simulink model "Main_System"  (R2024b)
settings: Solver=FixedStepAuto  StartTime=0.0  StopTime=10.0  FixedStep=0.01  RelTol=1e-3
model workspace (MAT data in the model file):
  U2 = Simulink.Parameter
  U2.Value = 1
  U2.Complexity = 'real'
  U2.Dimensions = [1 1]
  U2.DataType = 'auto'
  W = Simulink.Parameter
  W.Value = 10
  W.Complexity = 'real'
  W.Dimensions = [1 1]
  W.DataType = 'auto'
  W1 = Simulink.Parameter
  W1.Value = 8.71893412272
  W1.Complexity = 'real'
  W1.Dimensions = [1 1]
  W1.DataType = 'auto'
  W2 = Simulink.Parameter
  W2.Value = 4.12765808105
  W2.Complexity = 'real'
  W2.Dimensions = [1 1]
  W2.DataType = 'auto'
  mu1 = Simulink.Parameter
  mu1.Value = 0
  mu1.Complexity = 'real'
  mu1.Dimensions = [1 1]
  mu1.DataType = 'auto'
  mu2 = Simulink.Parameter
  mu2.Value = 0
  mu2.Complexity = 'real'
  mu2.Dimensions = [1 1]
  mu2.DataType = 'auto'
  pi = 3.142
  tou = Simulink.Parameter
  tou.Value = 5
  tou.Complexity = 'real'
  tou.Dimensions = [1 1]
  tou.DataType = 'auto'
  tou1 = Simulink.Parameter
  tou1.Value = 4.94300842285
  tou1.Complexity = 'real'
  tou1.Dimensions = [1 1]
  tou1.DataType = 'auto'
  tou2 = Simulink.Parameter
  tou2.Value = 4.95458272298
  tou2.Complexity = 'real'
  tou2.Dimensions = [1 1]
  tou2.DataType = 'auto'
settings Model: Creator=nith  LastModifiedBy=nith

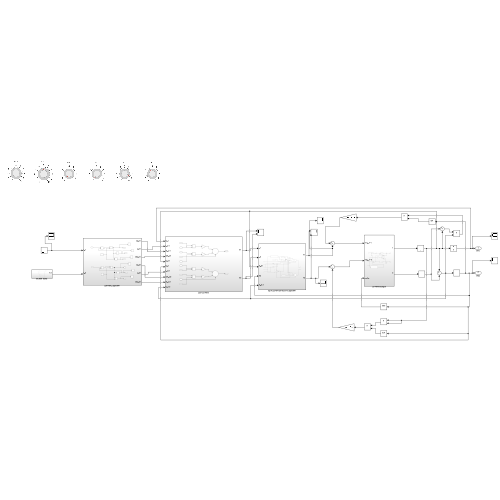
[thumbnail: Simulink's stored preview of the top-level diagram]
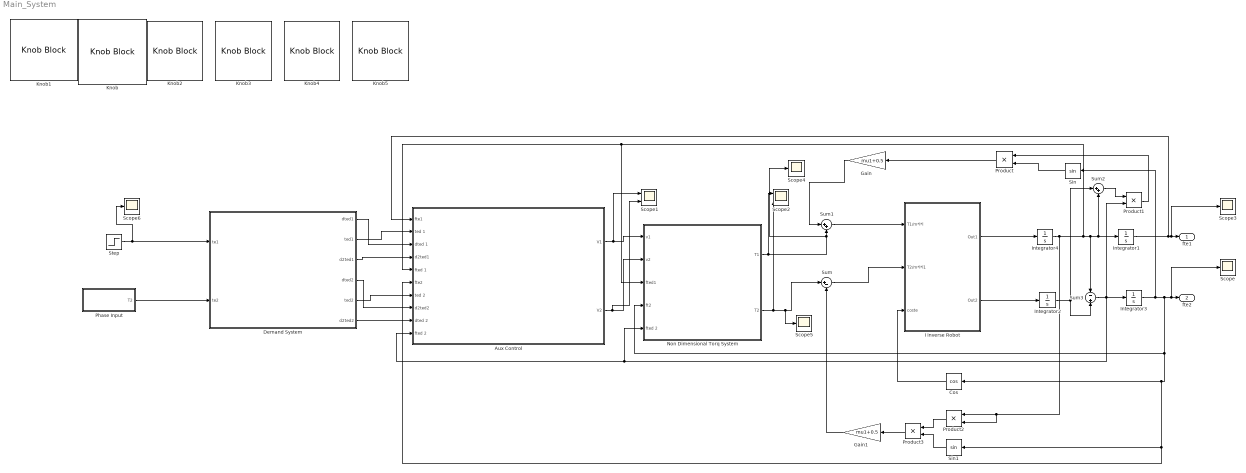
== system Main_System ==
  Aux Control : Subsystem
  Cos : Trigonometry  Operator=cos
  Demand System : Subsystem
  Gain : Gain  Gain=mu1+0.5
  Gain1 : Gain  Gain=mu1+0.5
  I inverse Robot : Subsystem
  Integrator{1..4} (4 alike) : Integrator
  Knob{,1..5} (6 alike) : KnobBlock  ScaleMax=10
  Non Dimensional Torq System : Subsystem
  Phase Input : Subsystem
  Product{,1..3} (4 alike) : Product
  Scope{,3..6} (5 alike) : Scope
  Scope1 : Scope  NumInputPorts=2
  Scope2 : Scope  NumInputPorts=2
  Sin : Trigonometry
  Sin1 : Trigonometry
  Step : Step  Time=0.5  After=6.87*(pi/180)  SampleTime=0
  Sum : Sum  Inputs=|+-
  Sum1 : Sum  Inputs=|++
  Sum2 : Sum  Inputs=|++
  Sum3 : Sum  Inputs=-+
  fte1 : Outport
  fte2 : Outport  Port=2
  wires:
  Demand System/2(ted1) -> Aux Control/2(ted 1)
  Demand System/1(dted1) -> Aux Control/3(dted 1)
  Demand System/3(d2ted1) -> Aux Control/4(d2ted1)
  Demand System/4(dted2) -> Aux Control/8(d2ted2)
  Demand System/5(ted2) -> Aux Control/7(ted 2)
  Demand System/6(d2ted2) -> Aux Control/9(dted 2)
  Integrator4/1 -> Sum3/1, Integrator1/1, Sum2/2, Non Dimensional Torq System/3(fted1), Aux Control/5(fted 1), Product2/2, Product2/1
  Integrator1/1 -> Aux Control/1(fte1), Scope3/1, fte1/1
  Integrator2/1 -> Sum2/1, Sum3/2
  Sum3/1 -> Non Dimensional Torq System/5(fted 2), Aux Control/10(fted 2), Integrator3/1, Product1/2
  Integrator3/1 -> Sin/1, Non Dimensional Torq System/4(ft2), Cos/1, Aux Control/6(fte2), Sin1/1, Scope/1, fte2/1
  Non Dimensional Torq System/1(T1) -> Scope2/1, Scope4/1, Sum1/2
  Non Dimensional Torq System/2(T2) -> Scope5/1, Sum/1, Scope2/2
  Sum1/1 -> I inverse Robot/1(T1/m*l*l)
  Sum/1 -> I inverse Robot/2(T2/m*l*l1)
  Cos/1 -> I inverse Robot/3(coste)
  Product2/1 -> Product3/1
  Sin1/1 -> Product3/2
  Sin/1 -> Product/2
  Product1/1 -> Product/1
  Sum2/1 -> Product1/1
  Aux Control/1(V1) -> Scope1/1, Non Dimensional Torq System/1(v1)
  Aux Control/2(V2) -> Scope1/2, Non Dimensional Torq System/2(v2)
  Product/1 -> Gain/1
  I inverse Robot/1(Out1) -> Integrator4/1
  I inverse Robot/2(Out2) -> Integrator2/1
  Phase Input/1(T2) -> Demand System/2(te2)
  Step/1 -> Scope6/1, Demand System/1(te1)
  Gain/1 -> Sum1/1
  Product3/1 -> Gain1/1
  Gain1/1 -> Sum/2

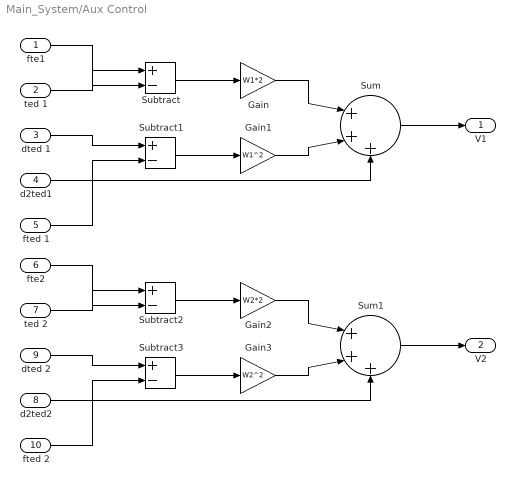
== system Main_System/Aux Control ==
  fte1 : Inport
  ted 1 : Inport  Port=2
  dted 1 : Inport  Port=3
  d2ted1 : Inport  Port=4
  fted 1 : Inport  Port=5
  fte2 : Inport  Port=6
  ted 2 : Inport  Port=7
  d2ted2 : Inport  Port=8
  dted 2 : Inport  Port=9
  fted 2 : Inport  Port=10
  Gain : Gain  Gain=W1*2
  Gain1 : Gain  Gain=W1^2
  Gain2 : Gain  Gain=W2*2
  Gain3 : Gain  Gain=W2^2
  Subtract{,1..3} (4 alike) : Sum  Inputs=+-
  Sum : Sum  Inputs=|+++
  Sum1 : Sum  Inputs=|+++
  V1 : Outport
  V2 : Outport  Port=2
  wires:
  Subtract/1 -> Gain/1
  Gain3/1 -> Sum1/2
  ted 2/1 -> Subtract2/1
  fted 2/1 -> Subtract3/2
  Sum/1 -> V1/1
  Sum1/1 -> V2/1
  dted 2/1 -> Subtract3/1
  fte1/1 -> Subtract/2
  Subtract3/1 -> Gain3/1
  d2ted1/1 -> Sum/3
  d2ted2/1 -> Sum1/3
  Gain/1 -> Sum/1
  Subtract1/1 -> Gain1/1
  Gain2/1 -> Sum1/1
  Gain1/1 -> Sum/2
  fte2/1 -> Subtract2/2
  ted 1/1 -> Subtract/1
  fted 1/1 -> Subtract1/2
  Subtract2/1 -> Gain2/1
  dted 1/1 -> Subtract1/1

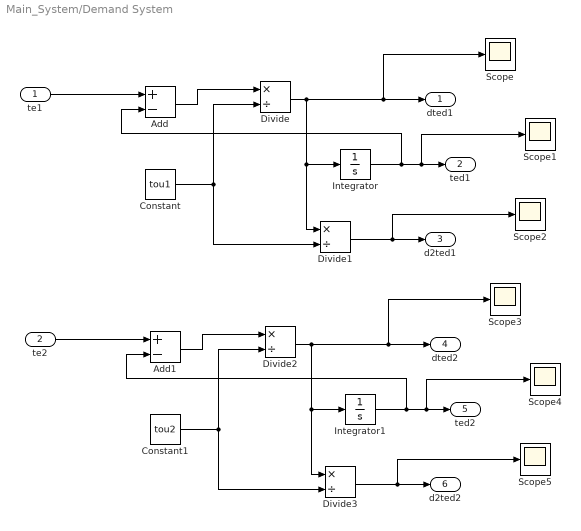
== system Main_System/Demand System ==
  te1 : Inport
  te2 : Inport  Port=2
  Add : Sum  Inputs=+-
  Add1 : Sum  Inputs=+-
  Constant : Constant  Value=tou1
  Constant1 : Constant  Value=tou2
  Divide{,1..3} (4 alike) : Product  Inputs=*/
  Integrator : Integrator
  Integrator1 : Integrator
  Scope{,1..5} (6 alike) : Scope
  dted1 : Outport
  ted1 : Outport  Port=2
  d2ted1 : Outport  Port=3
  dted2 : Outport  Port=4
  ted2 : Outport  Port=5
  d2ted2 : Outport  Port=6
  wires:
  Divide/1 -> Integrator/1, Divide1/1, Scope/1, dted1/1
  Integrator/1 -> Add/2, Scope1/1, ted1/1
  Constant/1 -> Divide1/2, Divide/2
  Divide1/1 -> Scope2/1, d2ted1/1
  te2/1 -> Add1/1
  Add/1 -> Divide/1
  Add1/1 -> Divide2/1
  Constant1/1 -> Divide3/2, Divide2/2
  Divide2/1 -> Integrator1/1, Divide3/1, Scope3/1, dted2/1
  te1/1 -> Add/1
  Integrator1/1 -> Add1/2, Scope4/1, ted2/1
  Divide3/1 -> Scope5/1, d2ted2/1

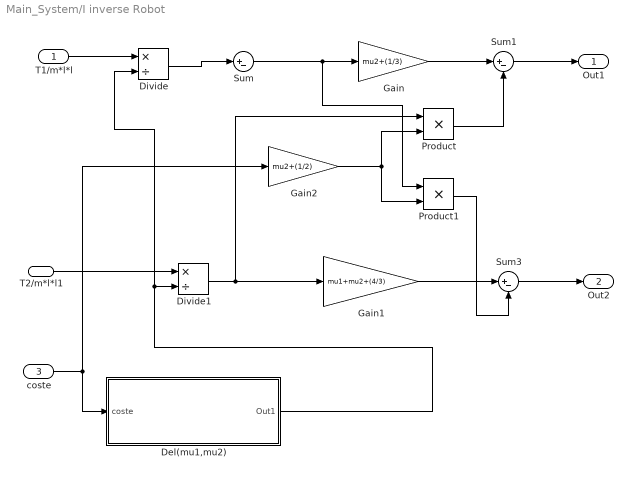
== system Main_System/I inverse Robot ==
  T1/m*l*l : Inport
  T2/m*l*l1 : Inport  Port=2
  coste : Inport  Port=3
  Del(mu1,mu2) : Subsystem
  Divide : Product  Inputs=*/
  Divide1 : Product  Inputs=*/
  Gain : Gain  Gain=mu2+(1/3)
  Gain1 : Gain  Gain=mu1+mu2+(4/3)
  Gain2 : Gain  Gain=mu2+(1/2)
  Product : Product
  Product1 : Product
  Sum : Sum  Inputs=|+-
  Sum1 : Sum  Inputs=|+-
  Sum3 : Sum  Inputs=|+-
  Out1 : Outport
  Out2 : Outport  Port=2
  wires:
  Sum/1 -> Product1/1, Gain/1
  T2/m*l*l1/1 -> Divide1/1
  Gain/1 -> Sum1/1
  Divide/1 -> Sum/1
  T1/m*l*l/1 -> Divide/1
  Sum1/1 -> Out1/1
  Del(mu1,mu2)/1(Out1) -> Divide/2, Divide1/2
  Gain2/1 -> Product1/2, Product/2
  coste/1 -> Del(mu1,mu2)/1(coste), Gain2/1
  Product/1 -> Sum1/2
  Divide1/1 -> Gain1/1, Product/1
  Sum3/1 -> Out2/1
  Gain1/1 -> Sum3/1
  Product1/1 -> Sum3/2

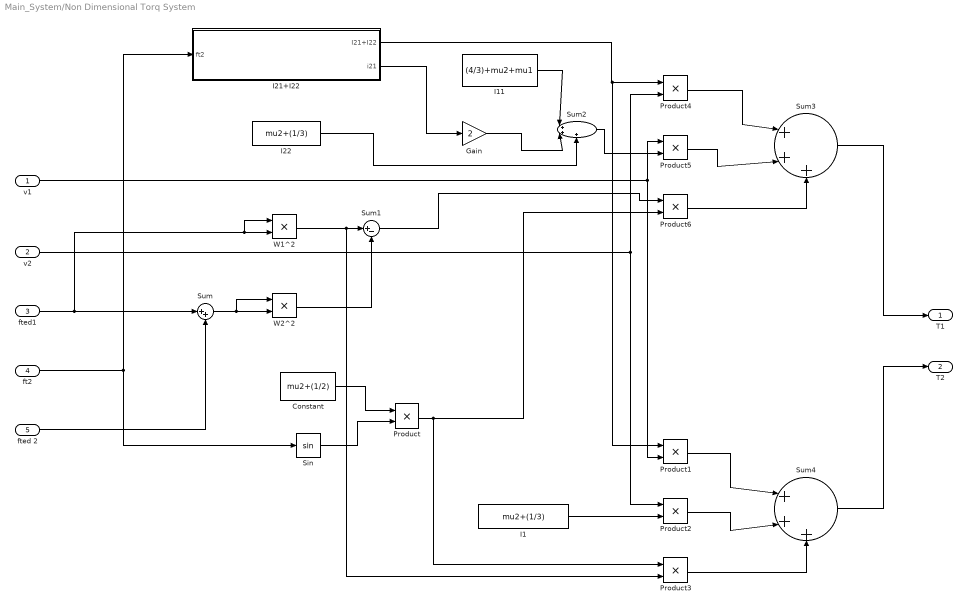
== system Main_System/Non Dimensional Torq System ==
  v1 : Inport
  v2 : Inport  Port=2
  fted1 : Inport  Port=3
  ft2 : Inport  Port=4
  fted 2 : Inport  Port=5
  Constant : Constant  Value=mu2+(1/2)
  Gain : Gain  Gain=2
  I1 : Constant  Value=mu2+(1/3)
  I11 : Constant  Value=(4/3)+mu2+mu1
  I21+I22 : Subsystem
  I22 : Constant  Value=mu2+(1/3)
  Product{,1..6} (7 alike) : Product
  Sin : Trigonometry
  Sum : Sum  Inputs=|++
  Sum1 : Sum  Inputs=|+-
  Sum2 : Sum  Inputs=|+++
  Sum3 : Sum  Inputs=|+++
  Sum4 : Sum  Inputs=|+++
  W1^2 : Product
  W2^2 : Product
  T1 : Outport
  T2 : Outport  Port=2
  wires:
  fted 2/1 -> Sum/2
  fted1/1 -> W1^2/1, W1^2/2, Sum/1
  Sum/1 -> W2^2/2, W2^2/1
  W1^2/1 -> Product3/2, Sum1/1
  W2^2/1 -> Sum1/2
  Constant/1 -> Product/1
  Sin/1 -> Product/2
  ft2/1 -> I21+I22/1(ft2), Sin/1
  Product/1 -> Product6/2, Product3/1
  I21+I22/2(i21) -> Gain/1
  I11/1 -> Sum2/1
  Gain/1 -> Sum2/2
  I22/1 -> Sum2/3
  Sum2/1 -> Product5/2
  I21+I22/1(I21+I22) -> Product1/1, Product4/1
  I1/1 -> Product2/2
  v1/1 -> Product1/2, Product5/1
  v2/1 -> Product2/1, Product4/2
  Sum1/1 -> Product6/1
  Product4/1 -> Sum3/1
  Product5/1 -> Sum3/2
  Product6/1 -> Sum3/3
  Product1/1 -> Sum4/1
  Product2/1 -> Sum4/2
  Product3/1 -> Sum4/3
  Sum4/1 -> T2/1
  Sum3/1 -> T1/1

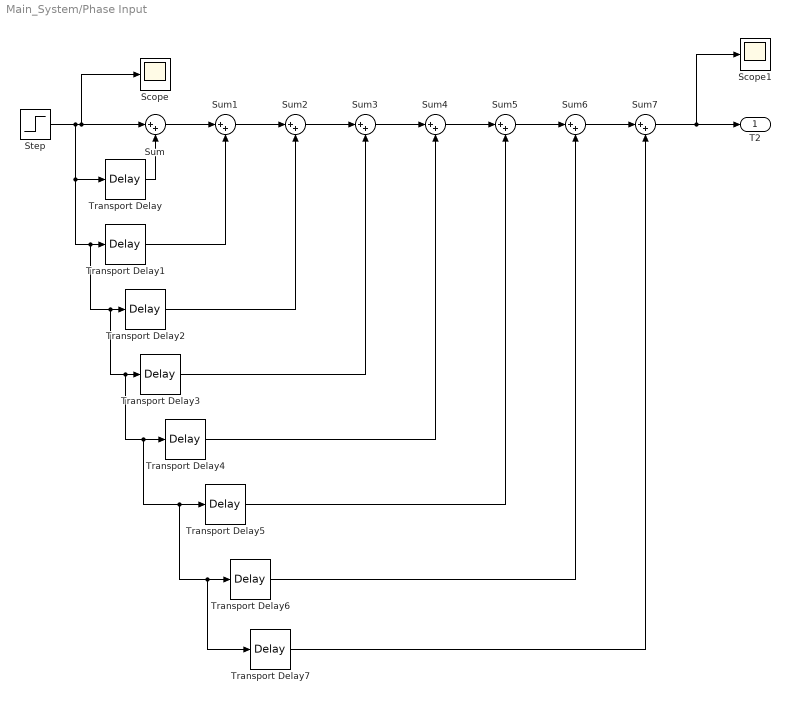
== system Main_System/Phase Input ==
  Scope : Scope
  Scope1 : Scope
  Step : Step  Time=0.5  After=pi/6  SampleTime=0
  Sum{,1..7} (8 alike) : Sum  Inputs=|++
  Transport Delay : TransportDelay
  Transport Delay1 : TransportDelay  DelayTime=2
  Transport Delay2 : TransportDelay  DelayTime=3
  Transport Delay3 : TransportDelay  DelayTime=4
  Transport Delay4 : TransportDelay  DelayTime=5
  Transport Delay5 : TransportDelay  DelayTime=6
  Transport Delay6 : TransportDelay  DelayTime=7
  Transport Delay7 : TransportDelay  DelayTime=8
  T2 : Outport
  wires:
  Transport Delay/1 -> Sum/2
  Step/1 -> Transport Delay7/1, Transport Delay6/1, Transport Delay5/1, Transport Delay4/1, Transport Delay3/1, Transport Delay2/1, Transport Delay1/1, Transport Delay/1, Scope/1, Sum/1
  Sum/1 -> Sum1/1
  Sum1/1 -> Sum2/1
  Sum4/1 -> Sum5/1
  Sum3/1 -> Sum4/1
  Sum2/1 -> Sum3/1
  Sum5/1 -> Sum6/1
  Transport Delay1/1 -> Sum1/2
  Transport Delay2/1 -> Sum2/2
  Transport Delay3/1 -> Sum3/2
  Transport Delay4/1 -> Sum4/2
  Transport Delay5/1 -> Sum5/2
  Transport Delay6/1 -> Sum6/2
  Transport Delay7/1 -> Sum7/2
  Sum6/1 -> Sum7/1
  Sum7/1 -> Scope1/1, T2/1

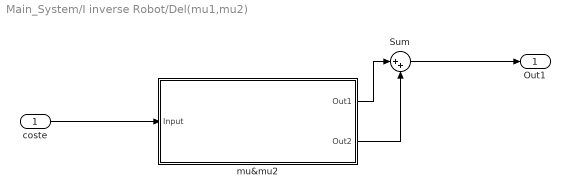
== system Main_System/I inverse Robot/Del(mu1,mu2) ==
  coste : Inport
  Sum : Sum  Inputs=|++
  mu&mu2 : Subsystem
  Out1 : Outport
  wires:
  mu&mu2/1(Out1) -> Sum/1
  mu&mu2/2(Out2) -> Sum/2
  coste/1 -> mu&mu2/1(Input)
  Sum/1 -> Out1/1

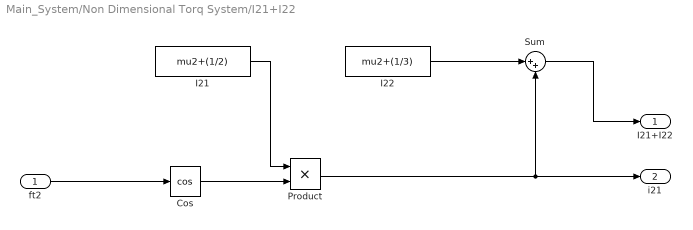
== system Main_System/Non Dimensional Torq System/I21+I22 ==
  ft2 : Inport
  Cos : Trigonometry  Operator=cos
  I21 : Constant  Value=mu2+(1/2)
  I22 : Constant  Value=mu2+(1/3)
  Product : Product
  Sum : Sum  Inputs=|++
  I21+I22 : Outport
  i21 : Outport  Port=2
  wires:
  ft2/1 -> Cos/1
  Cos/1 -> Product/2
  I21/1 -> Product/1
  I22/1 -> Sum/1
  Product/1 -> i21/1, Sum/2
  Sum/1 -> I21+I22/1

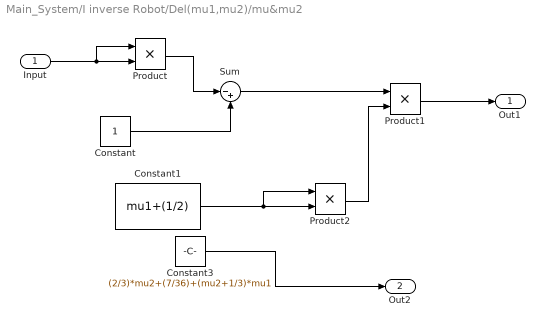
== system Main_System/I inverse Robot/Del(mu1,mu2)/mu&mu2 ==
  Input : Inport
  Constant : Constant
  Constant1 : Constant  Value=mu1+(1/2)
  Constant3 : Constant  Value=(2/3)*mu2+(7/36)+(mu2+1/3)*mu1
  Product : Product
  Product1 : Product
  Product2 : Product
  Sum : Sum  Inputs=|-+
  Out1 : Outport
  Out2 : Outport  Port=2
  wires:
  Input/1 -> Product/1, Product/2
  Product/1 -> Sum/1
  Constant/1 -> Sum/2
  Sum/1 -> Product1/1
  Constant1/1 -> Product2/2, Product2/1
  Product2/1 -> Product1/2
  Product1/1 -> Out1/1
  Constant3/1 -> Out2/1
